simulink model "mode_selection_test"  (R2016b)
settings: Solver=VariableStepAuto  StartTime=0.0  StopTime=6400  RelTol=1e-3
libraries: mode_selection x1
settings Model: Creator=Sean  LastModifiedBy=Sean

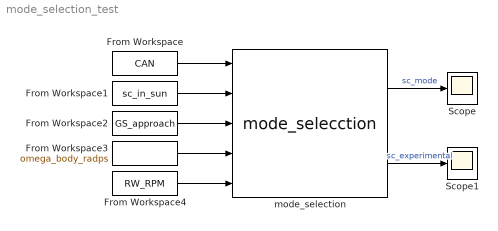
== system mode_selection_test ==
  From Workspace : FromWorkspace  VariableName=CAN  SampleTime=0
  From Workspace1 : FromWorkspace  VariableName=sc_in_sun  SampleTime=0
  From Workspace2 : FromWorkspace  VariableName=GS_approach  SampleTime=0
  From Workspace3 : FromWorkspace  VariableName=omega_body_radps  SampleTime=0
  From Workspace4 : FromWorkspace  VariableName=RW_RPM  SampleTime=0
  Scope : Scope
  Scope1 : Scope
  mode_selection : mode_selection/mode_selecction
  wires:
  mode_selection/1 -> Scope/1  "sc_mode"
  From Workspace1/1 -> mode_selection/2
  mode_selection/2 -> Scope1/1  "sc_experimental"
  From Workspace/1 -> mode_selection/1
  From Workspace2/1 -> mode_selection/3
  From Workspace3/1 -> mode_selection/4
  From Workspace4/1 -> mode_selection/5
